simulink model "fmtx_fm_fdm"  (R2014b)
settings: Solver=ode45  StartTime=0.0  StopTime=60  RelTol=1e-3
PreLoadFcn:
  | %%%%%%%%%%%%%%%%%%%%%%%%%%%%%%%%%%%%%%%%%%%%%%%%%%%%%%%%%%%%%%%%%%%%%%%%%%%
  | % check to see if Simulink library folder is missing from the MATLAB path %
  | %%%%%%%%%%%%%%%%%%%%%%%%%%%%%%%%%%%%%%%%%%%%%%%%%%%%%%%%%%%%%%%%%%%%%%%%%%%
  | if isempty(strfind(path, 'rtlsdr_book_library'))
  | 
  |     % create error window
  |     fig_error = figure(...
  |         'Name', 'Error: RTL-SDR Book Library',...
  |         'Toolbar','none',...
  |         'MenuBar','none',...
  |         'NumberTitle','off',...
  |         'Resize','off',...
  |         'WindowStyle','modal');
  |     fig_error.Position(3) = 600;
  |     fig_error.Position(4) = 150;
  |     fig_axes = axes(...
  |         'Parent',fig_error,...
  |         'Position',[0,0,1,1],...
  |         'visible','off');
  |     % error message
  |     t_title = text(.05,.8,...
  |         'MISSING DIRECTORIES',...
  |         'FontSize',11.5);
  |     t_body = text(.075,.6,...
  |         [{'Simulink cannot find the  \it{<root>}\rm / \it{rtlsdr\_book\_library}\rm  folder in the \it{MATLAB Path}\rm.'},...
  |         {'Please set the MATLAB path following the instructions given in Exercise 2.4.'}],...
  |         'FontSize',10.5);
  |     % buttons
  |     btn_path = uicontrol(...
  |         'Parent',fig_error,...
  |         'String','Set Path Now',...
  |         'FontSize',10,...
  |         'Callback', 'pathtool; close(fig_error);',...
  |         'Position', [fig_error.Position(3)/2-210, 30, 200, 30]);
  |     btn_abort = uicontrol(...
  |         'Parent',fig_error,...
  |         'String','No thanks',...
  |         'FontSize',10,...
  |         'Callback', 'close(fig_error); abort=1;',...
  |         'Position', [fig_error.Position(3)/2+10, 30, 200, 30]);
  | 
  |     % pause to allow user to interact with error box
  |     uiwait(fig_error);
  | 
  |     % abort simulation
  |     try
  |         if abort==1
  |             set_param(gcs, 'SimulationCommand', 'stop');
  |         end
  |     end
  | 
  |     % if user has set path, allow diagram to be updated
  |     if ~exist('abort','var')
  |         % create error window
  |         fig_update = figure(...
  |             'Name', 'Update Diagram',...
  |             'Toolbar','none',...
  |             'MenuBar','none',...
  |             'NumberTitle','off',...
  |             'Resize','off');
  | ... (+24 lines)
undefined symbols (not defined in the file): dfilt, fdesignblkfcn, gcbh
libraries: dsparch4 x6, dspvision x5, dspsrcs4 x2, rtlsdr_book_library x1
(part 2 of 2)

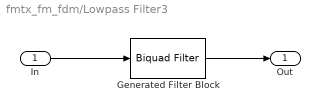
== system fmtx_fm_fdm/Lowpass Filter3 ==
  In : Inport
  Generated Filter Block : dsparch4/Biquad Filter  Tag=BlockMethodSubSystem  IIRFiltStruct=Direct form II  CoeffSource=Specify via dialog  BiQuadCoeffs=[0.02505658453151734 0.050113169063034681 0.02505658453151734 1 -1.6618358052504689 0.92327518660477159;0.037716014607021689 0.075432029214043378 0.037716014607021689 1 -1.5666197180702381 0.81307974054400167;0.048494542600695072 0.096989085201390143 0.048494542600695072 1 -1.483833787366122 0.71726995848240305;0.057562689362794101 0.1151253787255882 0.057562689362794101 1 -1.4124095756411101 0.63460931673938947;0.065066669960849324 0.13013333992169865 0.065066669960849324 1 -1.3513355886493104 0.5639271931762575;0.071126049882347511 0.14225209976469502 0.071126049882347511 1 -1.2996951874675289 0.50416274358054824;0.075826965263644491 0.15165393052728898 0.075826965263644491 1 -1.2566848480829704 0.45438603384519421;0.079207708097762716 0.15841541619552543 0.079207708097762716 1 -1.2216205877683222 0.41380547733850032;0.081213644661423695 0.16242728932284739 0.081213644661423695 1 -1.1939377721788489 0.38176761165383055;0.08148106483340975 0.1629621296668195 0.08148106483340975 1 -1.1731876770814522 0.35775311943117882;0.076637308661870573 0.15327461732374115 0.076637308661870573 1 -1.1590329311748637 0.34137155424355531;0.047546496662289287 0.095092993324578573 0.047546496662289287 1 -1.1512431451247189 0.3323562819935113;0.04540058431321875 0.090801168626437501 0.04540058431321875 1 -1.1496915016555413 0.3305605345596806;0.045831247000341468 0.091662494000682937 0.045831247000341468 1 -1.1543527405881076 0.3359550778409825;0.046516257123944797 0.093032514247889594 0.046516257123944797 1 -1.1653027462029997 0.34862773420436555;0.047466760014933662 0.094933520029867324 0.047466760014933662 1 -1.1827197756415799 0.36878480413735909;0.048698191344618065 0.09739638268923613 0.048698191344618065 1 -1.2068872094697505 0.39675424952948513;0.050230457593599342 0.10046091518719868 0.050230457593599342 1 -1.2381975142107695 0.43299027958924174;0.052088101393404251 0.1041762027868085 0.052088101393404251 1 -1.2771568309371673 0.47807866131156473;0.054300385989436643 0.10860077197887329 0.054300385989436643 1 -1.3243891792379572 0.53274158481157419;0.056901193140924844 0.11380238628184969 0.056901193140924844 1 -1.3806386047689676 0.59784014872671409;0.059928568932260555 0.11985713786452111 0.059928568932260555 1 -1.4467665832625731 0.6743713558262725;0.063423665332839996 0.12684733066567999 0.063423665332839996 1 -1.5237404723519465 0.76345474808098879;0.023993836801624483 0.047987673603248966 0.023993836801624483 1 -1.612606599730263 0.86630126106162297;0.014199710532717848 0.028399421065435696 0.014199710532717848 1 -1.7144385404499303 0.98415336424243371;0.028453803345255303 0.056907606690510606 0.028453803345255303 1 -1.6368075882726612 0.89430953998294882;0.04083171761385794 0.08166343522771588 0.04083171761385794 1 -1.5448001049050344 0.78782747407497666;0.051459392354549008 0.10291878470909802 0.051459392354549008 1 -1.4649534370622368 0.69541935859814075;0.060531990296125222 0.12106398059225044 0.060531990296125222 1 -1.3962083671487442 0.61585934024476119;0.06815377125244737 0.13630754250489474 0.06815377125244737 1 -1.3375744913620335 0.54800120526008977;0.074455848419753085 0.14891169683950617 0.074455848419753085 1 -1.2881623105057174 0.49081551877004753;0.079552479596548167 0.15910495919309633 0.079552479596548167 1 -1.2471979145071224 0.44340661946156557;0.083510197687583193 0.16702039537516639 0.083510197687583193 1 -1.2140273488611264 0.40501767295371627;0.086395360489223874 0.17279072097844775 0.086395360489223874 1 -1.1881153515668013 0.37502921002970635;0.08825814050628647 0.17651628101257294 0.08825814050628647 1 -1.1690414739763555 0.35295463721924042;0.072653340568011524 0.14530668113602305 0.072653340568011524 1 -1.1564954726095342 0.33843490365490059;0.10631278825624907 0.21262557651249814 0.10631278825624907 1 -1.150273121708774 0.33123365486006179;0.09066349956390464 0.09066349956390464 0 1 -0.57474884697500372 0;0.045700079748393248 0.091400159496786496 0.045700079748393248 1 -1.1526025576110279 ...(+1167 chars)Flag=Warning  IC=0  ICnum=0  ICden=0  InputProcessing=Columns as channels (frame based)  denAccumFracLength=30  denProdOutputFracLength=30  secondMemoryFracLength=15  roundingMode=Floor  overflowMode=off  ScaleValues=[0.038531123333914737;1;1;1;1;1;1;1;1;1;1;1;1;1;1;1;1;1;1;1;1;1;1;1;1;1;1;1;1;1;1;1;1;1;1;1;1;1;1;1;1;1;1;1;1;1;1;1;1;1;1]  optimizeScaleValues=off  ScaleValueMode=Specify via input port (g)  scaleValueFracLength=14  FilterSource=Specify via dialog  dfiltObjectName=dfilt.df2tsos([1 0.3 0.4],[1 0.1 0.2])
  Out : Outport
  wires:
  In/1 -> Generated Filter Block/1
  Generated Filter Block/1 -> Out/1

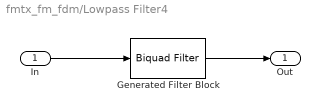
== system fmtx_fm_fdm/Lowpass Filter4 ==
  In : Inport
  Generated Filter Block : dsparch4/Biquad Filter  Tag=BlockMethodSubSystem  IIRFiltStruct=Direct form II  CoeffSource=Specify via dialog  BiQuadCoeffs=[0.02505658453151734 0.050113169063034681 0.02505658453151734 1 -1.6618358052504689 0.92327518660477159;0.037716014607021689 0.075432029214043378 0.037716014607021689 1 -1.5666197180702381 0.81307974054400167;0.048494542600695072 0.096989085201390143 0.048494542600695072 1 -1.483833787366122 0.71726995848240305;0.057562689362794101 0.1151253787255882 0.057562689362794101 1 -1.4124095756411101 0.63460931673938947;0.065066669960849324 0.13013333992169865 0.065066669960849324 1 -1.3513355886493104 0.5639271931762575;0.071126049882347511 0.14225209976469502 0.071126049882347511 1 -1.2996951874675289 0.50416274358054824;0.075826965263644491 0.15165393052728898 0.075826965263644491 1 -1.2566848480829704 0.45438603384519421;0.079207708097762716 0.15841541619552543 0.079207708097762716 1 -1.2216205877683222 0.41380547733850032;0.081213644661423695 0.16242728932284739 0.081213644661423695 1 -1.1939377721788489 0.38176761165383055;0.08148106483340975 0.1629621296668195 0.08148106483340975 1 -1.1731876770814522 0.35775311943117882;0.076637308661870573 0.15327461732374115 0.076637308661870573 1 -1.1590329311748637 0.34137155424355531;0.047546496662289287 0.095092993324578573 0.047546496662289287 1 -1.1512431451247189 0.3323562819935113;0.04540058431321875 0.090801168626437501 0.04540058431321875 1 -1.1496915016555413 0.3305605345596806;0.045831247000341468 0.091662494000682937 0.045831247000341468 1 -1.1543527405881076 0.3359550778409825;0.046516257123944797 0.093032514247889594 0.046516257123944797 1 -1.1653027462029997 0.34862773420436555;0.047466760014933662 0.094933520029867324 0.047466760014933662 1 -1.1827197756415799 0.36878480413735909;0.048698191344618065 0.09739638268923613 0.048698191344618065 1 -1.2068872094697505 0.39675424952948513;0.050230457593599342 0.10046091518719868 0.050230457593599342 1 -1.2381975142107695 0.43299027958924174;0.052088101393404251 0.1041762027868085 0.052088101393404251 1 -1.2771568309371673 0.47807866131156473;0.054300385989436643 0.10860077197887329 0.054300385989436643 1 -1.3243891792379572 0.53274158481157419;0.056901193140924844 0.11380238628184969 0.056901193140924844 1 -1.3806386047689676 0.59784014872671409;0.059928568932260555 0.11985713786452111 0.059928568932260555 1 -1.4467665832625731 0.6743713558262725;0.063423665332839996 0.12684733066567999 0.063423665332839996 1 -1.5237404723519465 0.76345474808098879;0.023993836801624483 0.047987673603248966 0.023993836801624483 1 -1.612606599730263 0.86630126106162297;0.014199710532717848 0.028399421065435696 0.014199710532717848 1 -1.7144385404499303 0.98415336424243371;0.028453803345255303 0.056907606690510606 0.028453803345255303 1 -1.6368075882726612 0.89430953998294882;0.04083171761385794 0.08166343522771588 0.04083171761385794 1 -1.5448001049050344 0.78782747407497666;0.051459392354549008 0.10291878470909802 0.051459392354549008 1 -1.4649534370622368 0.69541935859814075;0.060531990296125222 0.12106398059225044 0.060531990296125222 1 -1.3962083671487442 0.61585934024476119;0.06815377125244737 0.13630754250489474 0.06815377125244737 1 -1.3375744913620335 0.54800120526008977;0.074455848419753085 0.14891169683950617 0.074455848419753085 1 -1.2881623105057174 0.49081551877004753;0.079552479596548167 0.15910495919309633 0.079552479596548167 1 -1.2471979145071224 0.44340661946156557;0.083510197687583193 0.16702039537516639 0.083510197687583193 1 -1.2140273488611264 0.40501767295371627;0.086395360489223874 0.17279072097844775 0.086395360489223874 1 -1.1881153515668013 0.37502921002970635;0.08825814050628647 0.17651628101257294 0.08825814050628647 1 -1.1690414739763555 0.35295463721924042;0.072653340568011524 0.14530668113602305 0.072653340568011524 1 -1.1564954726095342 0.33843490365490059;0.10631278825624907 0.21262557651249814 0.10631278825624907 1 -1.150273121708774 0.33123365486006179;0.09066349956390464 0.09066349956390464 0 1 -0.57474884697500372 0;0.045700079748393248 0.091400159496786496 0.045700079748393248 1 -1.1526025576110279 ...(+1167 chars)Flag=Warning  IC=0  ICnum=0  ICden=0  InputProcessing=Columns as channels (frame based)  denAccumFracLength=30  denProdOutputFracLength=30  secondMemoryFracLength=15  roundingMode=Floor  overflowMode=off  ScaleValues=[0.038531123333914737;1;1;1;1;1;1;1;1;1;1;1;1;1;1;1;1;1;1;1;1;1;1;1;1;1;1;1;1;1;1;1;1;1;1;1;1;1;1;1;1;1;1;1;1;1;1;1;1;1;1]  optimizeScaleValues=off  ScaleValueMode=Specify via input port (g)  scaleValueFracLength=14  FilterSource=Specify via dialog  dfiltObjectName=dfilt.df2tsos([1 0.3 0.4],[1 0.1 0.2])
  Out : Outport
  wires:
  Generated Filter Block/1 -> Out/1
  In/1 -> Generated Filter Block/1
